simulink model "Sinus_yt"  (R2016b)
settings: Solver=VariableStepAuto  StartTime=0.0  StopTime=2  RelTol=1e-3
settings Model: Creator=live  LastModifiedBy=live

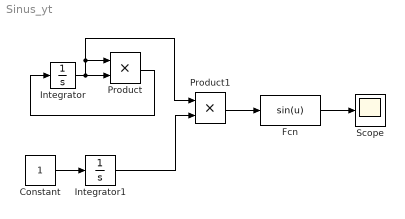
== system Sinus_yt ==
  Constant : Constant
  Fcn : Fcn  Expr=sin(u)
  Integrator : Integrator  InitialCondition=1
  Integrator1 : Integrator
  Product : Product
  Product1 : Product
  Scope : Scope
  wires:
  Integrator/1 -> Product1/1, Product/1, Product/2
  Product/1 -> Integrator/1
  Constant/1 -> Integrator1/1
  Integrator1/1 -> Product1/2
  Product1/1 -> Fcn/1
  Fcn/1 -> Scope/1
